simulink model "Hall_sensor_180deg"  (R2024b)
settings: Solver=ode15s  StartTime=0.0  StopTime=1.5  RelTol=1e-3
values from neighbouring files (symbols this model uses):
  control_mode = 1    [initialize_model.m]
  D_duty_cycle = 1e-3    (= 0.001)    [initialize_model.m]
  D_m = 1e-3    (= 0.001)    [initialize_model.m]
  hall_errors = [0 0 0]    [MTPA_sweep.m]    (also in initialize_model.m = (pi/180)*[-3,5,-4])
  I_duty_cycle = 1e-3    (= 0.001)    [initialize_model.m]
  J_t = 12e-4    (= 0.0012)    [initialize_model.m]
  L_ss = 0.45e-3    (= 0.00045)    [Arrow_86EMB3S98F_specs.m]    (also in M_2311P_specs.m = 0.0003657)
  lambda_m = 21.5e-3    (= 0.0215)    [Arrow_86EMB3S98F_specs.m]    (also in M_2311P_specs.m = 0.00985)
  P = 8    [Arrow_86EMB3S98F_specs.m]    (also in M_2311P_specs.m)
  P_duty_cycle = 10    [initialize_model.m]
  r_s = 0.15    [Arrow_86EMB3S98F_specs.m]    (also in M_2311P_specs.m = 0.345)
  T_m = torque_vals(i)    [MTPA_sweep.m]    (also in initialize_model.m = 1.53)
  tau_s = L_ss/r_s    (= 0.003)    [Arrow_86EMB3S98F_specs.m]    (also in M_2311P_specs.m = 0.00106)
  theta_v = pi/6    (= 0.523598775598)    [initialize_model.m]
  V_bus = 36    [initialize_model.m]
libraries: slpidlib x1, simulink x1, embmathops x1
settings Model: SimulationMode=accelerator  Creator=baolo  LastModifiedBy=baolo

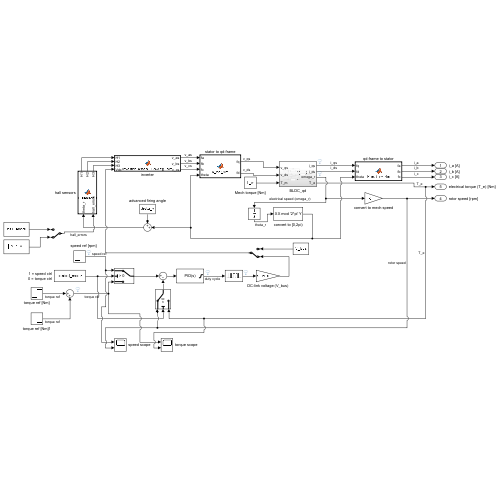
[thumbnail: Simulink's stored preview of the top-level diagram]
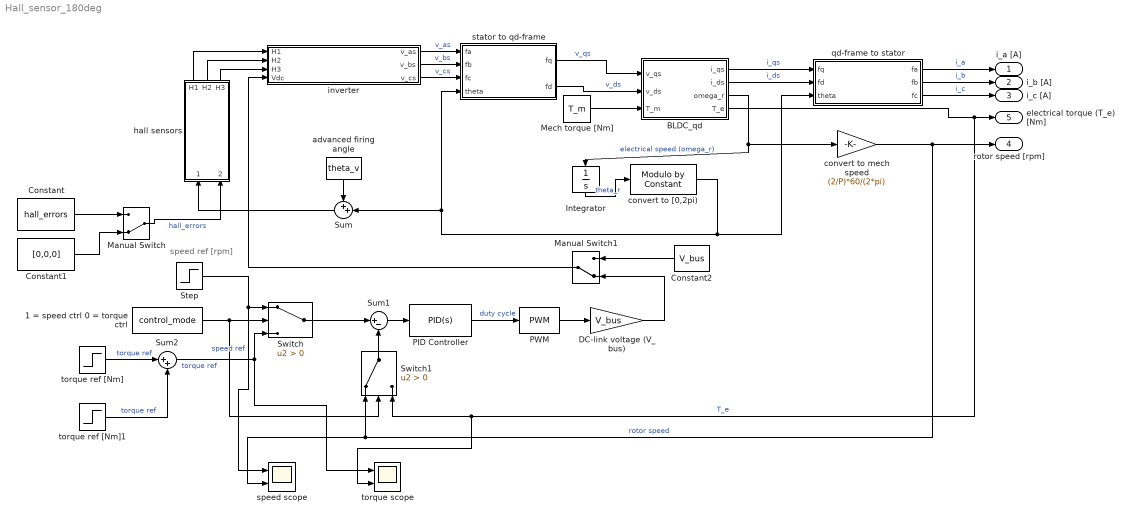
== system Hall_sensor_180deg ==
  note: speed ref [rpm]
  1 = speed ctrl 0 = torque ctrl : Constant  Value=control_mode
  BLDC_qd : Subsystem
  Constant : Constant  Value=hall_errors
  Constant1 : Constant  Value=[0,0,0]
  Constant2 : Constant  Value=V_bus
  DC-link voltage (V_bus) : Gain  Gain=V_bus
  Integrator : Integrator
  Manual Switch : ManualSwitch  CurrentSetting=0
  Manual Switch1 : ManualSwitch  CurrentSetting=0
  Mech torque [Nm] : Constant  Value=T_m
  PID Controller : slpidlib/PID Controller  Controller=PID  Form=Parallel  TimeDomain=Continuous-time  UseExternalTs=off  SampleTime=-1  IntegratorMethod=Forward Euler  FilterMethod=Forward Euler  ControllerParametersSource=internal  P=P_duty_cycle  I=I_duty_cycle  UseKiTs=off  D=D_duty_cycle  UseExternalDerivativeSource=off  N=100  UseFilter=on  TunerSelectOption=Transfer Function Based (PID Tuner App)  InitialConditionSource=internal  InitialConditionForIntegrator=0  InitialConditionForFilter=0  DifferentiatorICPrevScaledInput=0  ExternalReset=none  TrackingMode=off  Kt=1  LimitOutput=on  SatLimitsSource=internal  UpperSaturationLimit=1  LowerSaturationLimit=0  LinearizeAsGain=on  AntiWindupMode=none  Kb=1  LimitIntegrator=off  UpperIntegratorSaturationLimit=inf  LowerIntegratorSaturationLimit=-inf  POutMin=[]  POutMax=[]  IOutMin=[]  IOutMax=[]  DOutMin=[]  DOutMax=[]  NOutMin=[]  NOutMax=[]  SumOutMin=[]  SumOutMax=[]  SaturationOutMin=[]  SaturationOutMax=[]  PParamMin=[]  PParamMax=[]  IParamMin=[]  IParamMax=[]  DParamMin=[]  DParamMax=[]  NParamMin=[]  NParamMax=[]  KbParamMin=[]  KbParamMax=[]  KtParamMin=[]  KtParamMax=[]  KbOutMin=[]  KbOutMax=[]  KtOutMin=[]  KtOutMax=[]  IntegratorOutMin=[]  IntegratorOutMax=[]  FilterOutMin=[]  FilterOutMax=[]  SumI1OutMin=[]  SumI1OutMax=[]  SumI2OutMin=[]  SumI2OutMax=[]  SumI3OutMin=[]  SumI3OutMax=[]  SumI4OutMin=[]  SumI4OutMax=[]  SumDOutMin=[]  SumDOutMax=[]  DifferentiatorOutMin=[]  DifferentiatorOutMax=[]  FilterDiffOutCoefMin=[]  FilterDiffOutCoefMax=[]  ReciprocalOutMin=[]  ReciprocalOutMax=[]  SumDenOutMin=[]  SumDenOutMax=[]  SumNumOutMin=[]  SumNumOutMax=[]  DivideOutMin=[]  DivideOutMax=[]  UdiffTsProdOutMin=[]  UdiffTsProdOutMax=[]  NTsProdOutMin=[]  NTsProdOutMax=[]  UintegralTsProdOutMin=[]  UintegralTsProdOutMax=[]  UngainTsProdOutMin=[]  UngainTsProdOutMax=[]  ClampingZeroOutDataTypeStr=Inherit: Inherit via back propagation  ClampingZeroOutMin=[]  ClampingZeroOutMax=[]  FilterDenConstantOutDataTypeStr=Inherit: Inherit via back propagation  FilterDenConstantOutMin=[]  FilterDenConstantOutMax=[]  PCopyOutDataTypeStr=Inherit: Inherit via back propagation  PCopyOutMin=[]  PCopyOutMax=[]  NCopyOutDataTypeStr=Inherit: Inherit via back propagation  NCopyOutMin=[]  NCopyOutMax=[]  IntegratorContinuousStateAttributes=''  IntegratorStateMustResolveToSignalObject=off  IntegratorRTWStateStorageClass=Auto  FilterContinuousStateAttributes=''  FilterStateMustResolveToSignalObject=off  FilterRTWStateStorageClass=Auto  ParallelPVariant=InternalParameters  IdealPVariant=Disabled  IVariant=InternalParameters  DVariant=InternalParameters  IntegratorVariant=Continuous  SatVariant=Enabled  AWVariant=Passthrough  PCopyVariant=Disabled  TRVariant=Disabled  FdbkBlocksVariant=Forward  IdealPFdbkVariant=Disabled  SatFdbkVariant=Disabled  DerivativeFilterVariant=ContFilter  NVariant=InternalParameters  NCopyVariant=Disabled  FilterICVariant=InternalICsFilter  IntegratorICVariant=InternalICs  ExternalResetVariant=Disabled  TRSumVariant=Passthrough  SumFdbkVariant=Disabled  SumVariant=Sum_PID  TsampFilterVariant=InternalTs  TsampNgainVariant=Passthrough  TsampIntegralVariant=Disabled_SignalSpec  ExternalSaturationOutDataTypeStr=Inherit: Same as second input  DerivativeSourceVariant=ErrorSignal  PreIntVariant=InternalPreInt
  PWM : simulink/Discontinuities/PWM  DisableCoverage=on  Period=1/50000  InitialDelay=0  DisallowZeroDutyCycle=off  RunAtFixedTimeIntervals=off  SampleTime=0.1
  Step : Step  Time=0.1  After=1000  SampleTime=0
  Sum : Sum  Inputs=++|
  Sum1 : Sum  Inputs=|+-
  Sum2 : Sum  Inputs=|++
  Switch : Switch  Criteria=u2 > Threshold  SaturateOnIntegerOverflow=off  InputSameDT=off
  Switch1 : Switch  Criteria=u2 > Threshold  SaturateOnIntegerOverflow=off  InputSameDT=off
  advanced firing angle : Constant  Value=theta_v
  convert to [0,2pi) : embmathops/Modulo by Constant  Denominator=2*pi  SimulateUsing=Code generation
      settings: LibrarySourceBlock=embeddedMathLib/Modulo by Constant
  convert to mech speed : Gain  Gain=(2/P)*60/(2*pi)
  hall sensors : MATLAB Function  TreatAsAtomicUnit=on
  inverter : MATLAB Function  TreatAsAtomicUnit=on
  qd-frame to stator : MATLAB Function  TreatAsAtomicUnit=on
  speed scope : Scope  NumInputPorts=2
  stator to qd-frame : MATLAB Function  TreatAsAtomicUnit=on
  torque ref [Nm] : Step  Time=0.1  After=1e-1  SampleTime=0  ZeroCross=off
  torque ref [Nm]1 : Step  After=-0.5e-1  SampleTime=0
  torque scope : Scope  NumInputPorts=2
  i_a [A] : Outport
  i_b [A] : Outport  Port=2
  i_c [A] : Outport  Port=3
  rotor speed [rpm] : Outport  Port=4
  electrical torque (T_e) [Nm] : Outport  Port=5
  wires:
  stator to qd-frame/1(fq) -> BLDC_qd/1(v_qs)  "v_qs"
  stator to qd-frame/2(fd) -> BLDC_qd/2(v_ds)  "v_ds"
  Mech torque [Nm]/1 -> BLDC_qd/3(T_m)
  BLDC_qd/1(i_qs) -> qd-frame to stator/1(fq)  "i_qs"
  BLDC_qd/2(i_ds) -> qd-frame to stator/2(fd)  "i_ds"
  BLDC_qd/3(omega_r) -> convert to mech speed/1, Integrator/1  "electrical speed (omega_r)"
  convert to [0,2pi)/1 -> stator to qd-frame/4(theta), Sum/2, qd-frame to stator/3(theta)
  inverter/1(v_as) -> stator to qd-frame/1(fa)  "v_as"
  inverter/2(v_bs) -> stator to qd-frame/2(fb)  "v_bs"
  inverter/3(v_cs) -> stator to qd-frame/3(fc)  "v_cs"
  Integrator/1 -> convert to [0,2pi)/1  "theta_r"
  hall sensors/1(H1) -> inverter/1(H1)
  hall sensors/2(H2) -> inverter/2(H2)
  hall sensors/3(H3) -> inverter/3(H3)
  advanced firing angle/1 -> Sum/1
  Sum/1 -> hall sensors/1(theta_r)
  qd-frame to stator/1(fa) -> i_a [A]/1  "i_a"
  qd-frame to stator/2(fb) -> i_b [A]/1  "i_b"
  qd-frame to stator/3(fc) -> i_c [A]/1  "i_c"
  convert to mech speed/1 -> rotor speed [rpm]/1, speed scope/2, Switch1/1  "rotor speed"
  BLDC_qd/4(T_e) -> torque scope/2, Switch1/3, electrical torque (T_e) [Nm]/1  "T_e"
  1 = speed ctrl 0 = torque ctrl/1 -> Switch/2, Switch1/2
  Step/1 -> speed scope/1, Switch/1  "speed ref"
  Sum2/1 -> torque scope/1, Switch/3  "torque ref"
  Switch1/1 -> Sum1/2
  Switch/1 -> Sum1/1
  Sum1/1 -> PID Controller/1
  PID Controller/1 -> PWM/1  "duty cycle"
  PWM/1 -> DC-link voltage (V_bus)/1
  torque ref [Nm]/1 -> Sum2/1  "torque ref"
  torque ref [Nm]1/1 -> Sum2/2  "torque ref"
  Constant/1 -> Manual Switch/1
  Manual Switch/1 -> hall sensors/2(hall_errors)  "hall_errors"
  Constant1/1 -> Manual Switch/2
  Manual Switch1/1 -> inverter/4(Vdc)
  DC-link voltage (V_bus)/1 -> Manual Switch1/2
  Constant2/1 -> Manual Switch1/1

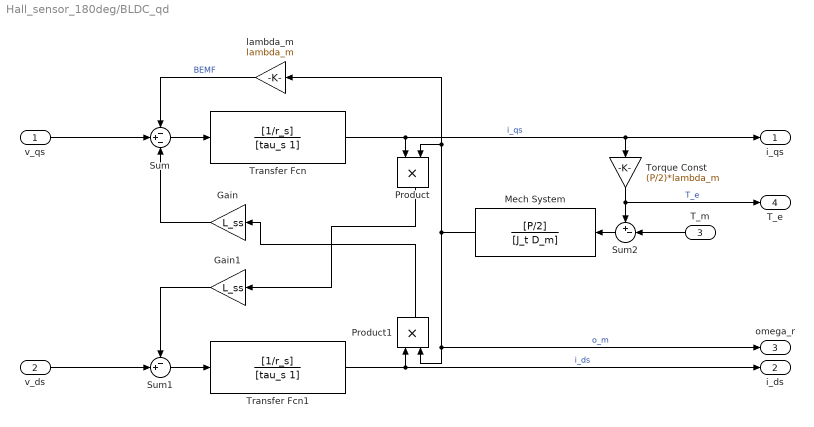
== system Hall_sensor_180deg/BLDC_qd ==
  v_qs : Inport
  v_ds : Inport  Port=2
  T_m : Inport  Port=3
  Gain : Gain  Gain=L_ss
  Gain1 : Gain  Gain=L_ss
  Mech System : TransferFcn  Numerator=[P/2]  Denominator=[J_t D_m]
  Product : Product
  Product1 : Product
  Sum : Sum  Inputs=-+-
  Sum1 : Sum  Inputs=-+|
  Sum2 : Sum  Inputs=+-|
  Torque Const : Gain  Gain=(P/2)*lambda_m
  Transfer Fcn : TransferFcn  Numerator=[1/r_s]  Denominator=[tau_s 1]
  Transfer Fcn1 : TransferFcn  Numerator=[1/r_s]  Denominator=[tau_s 1]
  lambda_m : Gain  Gain=lambda_m
  i_qs : Outport
  i_ds : Outport  Port=2
  omega_r : Outport  Port=3
  T_e : Outport  Port=4
  wires:
  T_m/1 -> Sum2/2
  Sum1/1 -> Transfer Fcn1/1
  Gain1/1 -> Sum1/1
  Product1/1 -> Gain/1
  Transfer Fcn1/1 -> i_ds/1, Product1/1  "i_ds"
  Mech System/1 -> lambda_m/1, Product/2, omega_r/1, Product1/2  "o_m"
  Torque Const/1 -> T_e/1, Sum2/1  "T_e"
  v_ds/1 -> Sum1/2
  Transfer Fcn/1 -> i_qs/1, Torque Const/1, Product/1  "i_qs"
  Product/1 -> Gain1/1
  Gain/1 -> Sum/3
  v_qs/1 -> Sum/2
  Sum/1 -> Transfer Fcn/1
  Sum2/1 -> Mech System/1
  lambda_m/1 -> Sum/1  "BEMF"

== matlab function Hall_sensor_180deg/qd-frame to stator ==
  data: fa output; fb output; fc output; fq input; fd input; theta input
function [fa,fb,fc] = K_mat_inv_sim(fq,fd,theta)
[fa,fb,fc] = K_mat_inv(fq,fd,theta);

== matlab function Hall_sensor_180deg/stator to qd-frame ==
  data: fa input; fq output; fb input; fc input; theta input; fd output
function [fq,fd] = K_mat_sim(fa,fb,fc,theta)
[fq,fd] = K_mat(fa,fb,fc,theta);

== matlab function Hall_sensor_180deg/inverter ==
  data: H1 input; v_as output; H2 input; H3 input; Vdc input; v_bs output; v_cs output
function [v_as, v_bs, v_cs] = inverter_6step_120deg_sim(H1,H2,H3,Vdc)
[v_as, v_bs, v_cs] = inverter_6step_180deg(H1,H2,H3, Vdc);
end

== matlab function Hall_sensor_180deg/hall sensors ==
  data: theta_r input; H1 output; H2 output; H3 output; hall_errors input
function [H1,H2,H3] = hall_sensor_sim(theta_r, hall_errors)
[H1,H2,H3] = hall_sensor(theta_r, hall_errors);
end
